simulink model "Mathematics_QuaternionDerivative_TH"  (Simulink 7.8)
settings: Solver=ode4  StartTime=0.0  StopTime=72  FixedStep=0.1  RelTol=1e-3
libraries: simulink_extras x2, AeroSim x2, aerolibtransform2 x1
settings Model: Creator=Ryan  LastModifiedBy=Ryan

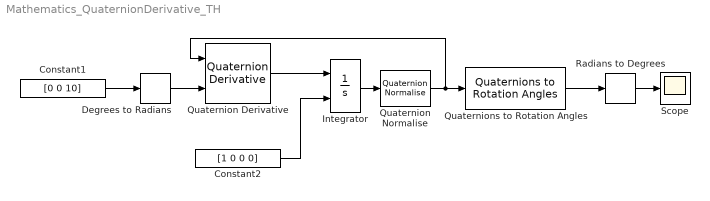
== system Mathematics_QuaternionDerivative_TH ==
  Constant1 : Constant  Value=[0 0 10]
  Constant2 : Constant  Value=[1 0 0 0]
  Degrees to Radians : simulink_extras/Transformations/Degrees to Radians
  Integrator : Integrator  InitialConditionSource=external
  Quaternion Derivative : AeroSim/Mathematics/Quaternion Derivative
  Quaternion Normalise : AeroSim/Mathematics/Quaternion Normalise
  Quaternions to Rotation Angles : aerolibtransform2/Quaternions to Rotation Angles  rotationOrder=ZYX
  Radians to Degrees : simulink_extras/Transformations/Radians to Degrees
  Scope : Scope
  wires:
  Constant1/1 -> Degrees to Radians/1
  Degrees to Radians/1 -> Quaternion Derivative/2
  Quaternion Derivative/1 -> Integrator/1
  Constant2/1 -> Integrator/2
  Integrator/1 -> Quaternion Normalise/1
  Quaternions to Rotation Angles/1 -> Radians to Degrees/1
  Radians to Degrees/1 -> Scope/1
  Quaternion Normalise/1 -> Quaternions to Rotation Angles/1, Quaternion Derivative/1
